simulink subsystem "VehicleBody3DOFLongitudinal"  (R2025b)
settings: Solver=VariableStepAuto  StartTime=0.0  StopTime=10.0  RelTol=1e-3
undefined symbols (not defined in the file): EnvAirTemp, EnvGrvty, PlntVehCGHgtAxl, PlntVehDstCGRearAxl, PlntVehHtchDst, PlntVehHtchHgtAxl, PlntVehHtchLatDst, PlntVehInitVertPos, PlntVehMass
libraries: autolibshared x1
settings Model: ModifiedByFormat=The MathWorks, Inc.  Creator=The MathWorks, Inc.  LastModifiedBy=The MathWorks, Inc.
settings OptimizationCC: ReuseModelBlockBuffer=off
settings DebuggingCC: SubsystemReferenceDiagnosticForUnitTest=warning
settings RTWCC: GPUComputeCapability=3.5

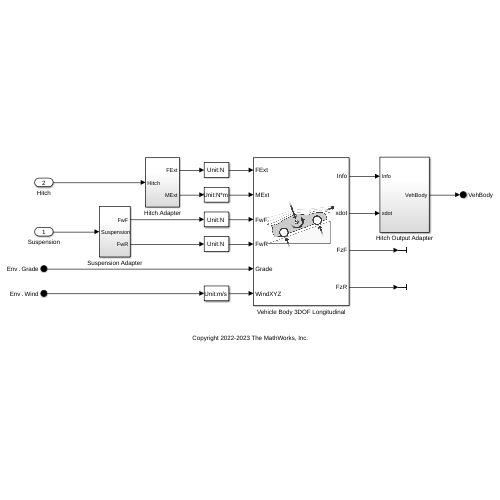
[thumbnail: Simulink's stored preview of the top-level diagram]
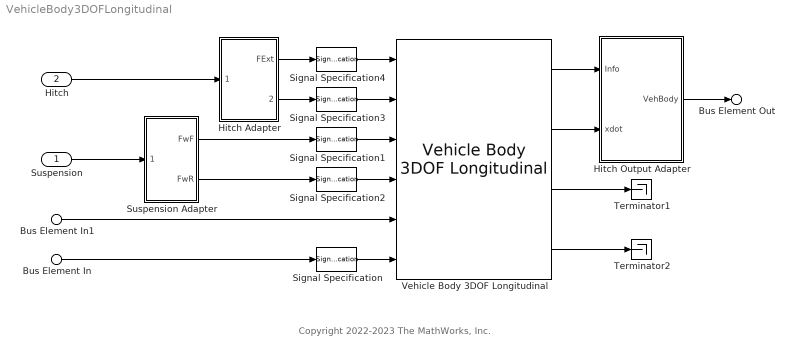
== system VehicleBody3DOFLongitudinal ==
  note: Copyright 2022-2023 The MathWorks, Inc.
  Suspension : Inport
  Hitch : Inport  Port=2
  Bus Element In : Inport  Port=3  PortName=Env  Element=Wind
  Bus Element In1 : Inport  Port=3  PortName=Env  Element=Grade
  Hitch Adapter : Subsystem
  Hitch Output Adapter : Subsystem
  Signal Specification : SignalSpecification  Unit=m/s
  Signal Specification1 : SignalSpecification  Unit=N
  Signal Specification2 : SignalSpecification  Unit=N
  Signal Specification3 : SignalSpecification  Unit=N*m
  Signal Specification4 : SignalSpecification  Unit=N
  Suspension Adapter : Subsystem
  Terminator1 : Terminator
  Terminator2 : Terminator
  Vehicle Body 3DOF Longitudinal : autolibshared/Vehicle Body 3DOF Longitudinal  VariantControl=SL  groundType=Grade angle  aMode=6  extFMode=on  extMMode=on  extTamb=off  NF=PlntVehNumWhlFrntAxl  NR=PlntVehNumWhlRearAxl  m=PlntVehMass  a=PlntVehDstCGFrntAxl  b=PlntVehDstCGRearAxl  h=PlntVehCGHgtAxl  Cd=PlntVehAeroDragCff  Af=PlntVehAeroFrntArea  x_o=PlntVehInitLongPos  xdot_o=PlntVehInitLongVel  Cl=PlntVehAeroLiftCff  z_o=PlntVehInitVertPos-PlntVehCGHgtAxl  zdot_o=0  Iyy=PlntVehPitchMomentInertia  Cpm=PlntVehAeroPitchCff  theta_o=0  q_o=0  FskF=[-50, -1, 0, 2, 3, 52].*1.5e4  dzsF=[-5e-3, -1e-4, 0, .2, .2001, .2051]  FsbF=[-10000 -100 -10 0 10 100 10000]*10  dzdotsF=[-10 -1 -.1 0 .1 1 10]  FskR=[-50, -1, 0, 2, 3, 52].*1e4  dzsR=[-5e-3, -1e-4, 0, .2, .2001, .2051]  FsbR=[-10000 -100 -10 0 10 100 10000]*10  dzdotsR=[-10 -1 -.1 0 .1 1 10]  Pabs=EnvAbsPrs  T=EnvAirTemp  g=EnvGrvty  blkID=0
  Bus Element Out : Outport  PortName=VehBody
  wires:
  Hitch/1 -> Hitch Adapter/1(Hitch)
  Suspension Adapter/2(FwR) -> Signal Specification2/1
  Hitch Adapter/2(MExt) -> Signal Specification3/1
  Hitch Adapter/1(FExt) -> Signal Specification4/1
  Suspension/1 -> Suspension Adapter/1(Suspension)
  Suspension Adapter/1(FwF) -> Signal Specification1/1
  Signal Specification3/1 -> Vehicle Body 3DOF Longitudinal/2
  Signal Specification4/1 -> Vehicle Body 3DOF Longitudinal/1
  Bus Element In/1 -> Signal Specification/1
  Vehicle Body 3DOF Longitudinal/1 -> Hitch Output Adapter/1(Info)
  Vehicle Body 3DOF Longitudinal/3 -> Terminator1/1
  Vehicle Body 3DOF Longitudinal/4 -> Terminator2/1
  Signal Specification/1 -> Vehicle Body 3DOF Longitudinal/6
  Bus Element In1/1 -> Vehicle Body 3DOF Longitudinal/5
  Signal Specification1/1 -> Vehicle Body 3DOF Longitudinal/3
  Signal Specification2/1 -> Vehicle Body 3DOF Longitudinal/4
  Hitch Output Adapter/1(VehBody) -> Bus Element Out/1
  Vehicle Body 3DOF Longitudinal/2 -> Hitch Output Adapter/2(xdot)

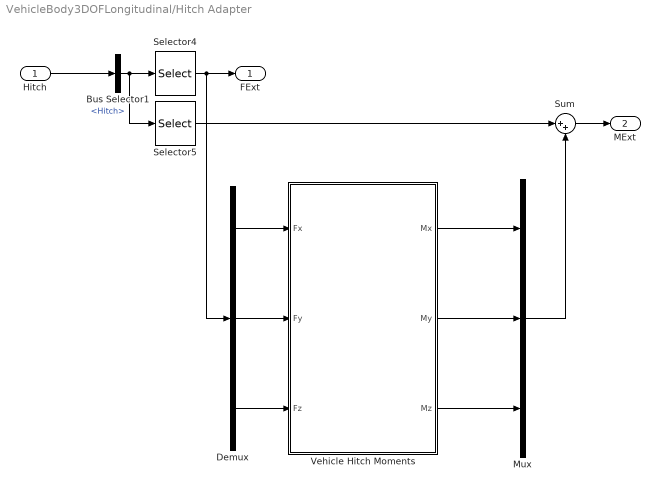
== system VehicleBody3DOFLongitudinal/Hitch Adapter ==
  Hitch : Inport
  Bus Selector1 : BusSelector  OutputSignals=Hitch
  Demux : Demux  Outputs=3
  Mux : Mux  Inputs=3
  Selector4 : Selector  InputPortWidth=6  IndexOptions=Index vector (dialog)  Indices=[1:3]  OutputSizes=1
  Selector5 : Selector  InputPortWidth=6  IndexOptions=Index vector (dialog)  Indices=[4:6]  OutputSizes=1
  Sum : Sum  Inputs=|++
  Vehicle Hitch Moments : Subsystem  mask{h=PlntVehCGHgtAxl, dh=PlntVehHtchDst, hh=PlntVehHtchHgtAxl, hl=PlntVehHtchLatDst}
      mask prompts: h "vdynblks:vehdynTractorBody6Dof:blkPrm_h"; dh "vdynblks:vehdynTractorBody6Dof:blkPrm_dh"; hh "vdynblks:vehdynTractorBody6Dof:blkPrm_hh"; hl "vdynblks:vehdynTractorBody6Dof:blkPrm_hl"
      mask DialogControl h Prompt: Vertical distance from center of mass to axle plane, h [m]:
      mask DialogControl dh Prompt: Longitudinal distance from center of mass to hitch, dh [m]:
      mask DialogControl hh Prompt: Vertical distance from hitch to axle plane, hh [m]:
      mask DialogControl hl Prompt: Lateral distance from geometric centerline to hitch, hl [m]:
  FExt : Outport
  MExt : Outport  Port=2
  wires:
  Selector5/1 -> Sum/1
  Bus Selector1/1 -> Selector5/1, Selector4/1  "<Hitch>"
  Selector4/1 -> FExt/1, Demux/1
  Hitch/1 -> Bus Selector1/1
  Demux/1 -> Vehicle Hitch Moments/1(Fx)
  Demux/2 -> Vehicle Hitch Moments/2(Fy)
  Demux/3 -> Vehicle Hitch Moments/3(Fz)
  Vehicle Hitch Moments/1(Mx) -> Mux/1
  Vehicle Hitch Moments/2(My) -> Mux/2
  Vehicle Hitch Moments/3(Mz) -> Mux/3
  Sum/1 -> MExt/1
  Mux/1 -> Sum/2

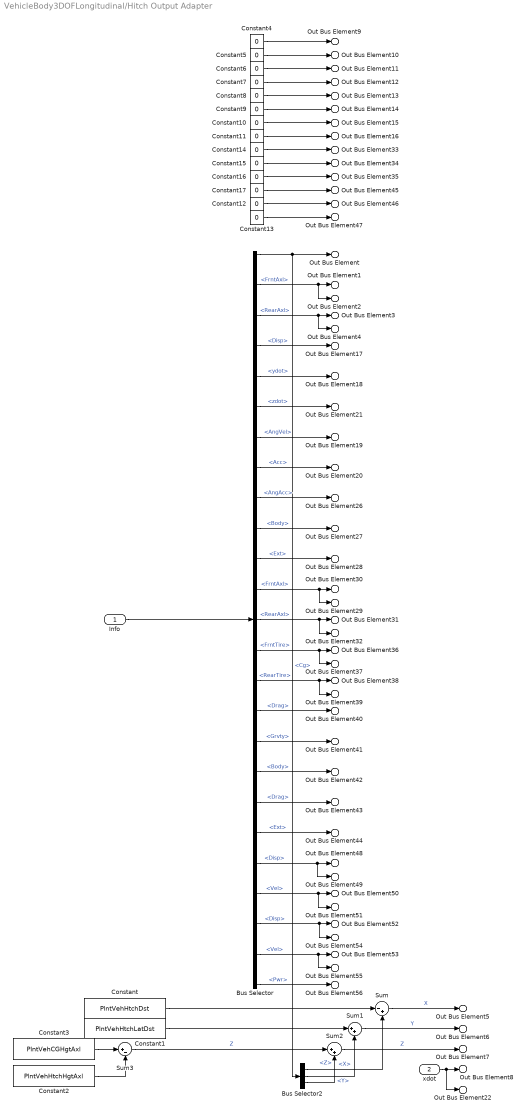
== system VehicleBody3DOFLongitudinal/Hitch Output Adapter ==
  Info : Inport
  xdot : Inport  Port=2
  Bus Selector : BusSelector  OutputSignals=InertFrm.Cg,InertFrm.FrntAxl,InertFrm.RearAxl,BdyFrm.Cg.Disp,BdyFrm.Cg.Vel.ydot,BdyFrm.Cg.Vel.zdot,BdyFrm.Cg.AngVel,BdyFrm.Cg.Acc,BdyFrm.Cg.AngAcc,BdyFrm.Forces.Body,BdyFrm.Forces.Ext,BdyFrm.Forces.FrntAxl,BdyFrm.Forces.RearAxl,BdyFrm.Forces.Tires.FrntTire,BdyFrm.Forces.Tires.RearTire,BdyFrm.Forces.Drag,BdyFrm.Forces.Grvty,BdyFrm.Moments.Body,BdyFrm.Moments.Drag,BdyFrm.Moments.Ext,BdyFrm.FrntAxl.Disp,BdyFrm.FrntAxl.Vel,BdyFrm.RearAxl.Disp,BdyFrm.RearAxl.Vel,BdyFrm.Pwr
  Bus Selector2 : BusSelector  OutputSignals=Disp.X,Disp.Y,Disp.Z
  Constant : Constant  Value=PlntVehHtchDst  SampleTime=-1
  Constant1 : Constant  Value=PlntVehHtchLatDst  SampleTime=-1
  Constant{4..17} (14 alike) : Constant  Value=0  SampleTime=-1
  Constant2 : Constant  Value=PlntVehHtchHgtAxl  SampleTime=-1
  Constant3 : Constant  Value=PlntVehCGHgtAxl  SampleTime=-1
  Sum : Sum  Inputs=|-+
  Sum1 : Sum  Inputs=|++
  Sum2 : Sum  Inputs=|++
  Sum3 : Sum  Inputs=|+-
  Out Bus Element : Outport  PortName=VehBody  Element=InertFrm.Cg
  Out Bus Element1 : Outport  PortName=VehBody  Element=InertFrm.FrntAxl.Lft
  Out Bus Element2 : Outport  PortName=VehBody  Element=InertFrm.FrntAxl.Rght
  Out Bus Element3 : Outport  PortName=VehBody  Element=InertFrm.RearAxl.Lft
  Out Bus Element4 : Outport  PortName=VehBody  Element=InertFrm.RearAxl.Rght
  Out Bus Element5 : Outport  PortName=VehBody  Element=InertFrm.Hitch.Disp.X
  Out Bus Element6 : Outport  PortName=VehBody  Element=InertFrm.Hitch.Disp.Y
  Out Bus Element7 : Outport  PortName=VehBody  Element=InertFrm.Hitch.Disp.Z
  Out Bus Element8 : Outport  PortName=VehBody  Element=InertFrm.Hitch.Vel.Xdot
  Out Bus Element9 : Outport  PortName=VehBody  Element=InertFrm.Hitch.Vel.Ydot
  Out Bus Element10 : Outport  PortName=VehBody  Element=InertFrm.Hitch.Vel.Zdot
  Out Bus Element11 : Outport  PortName=VehBody  Element=InertFrm.Geom.Disp.X
  Out Bus Element12 : Outport  PortName=VehBody  Element=InertFrm.Geom.Disp.Y
  Out Bus Element13 : Outport  PortName=VehBody  Element=InertFrm.Geom.Disp.Z
  Out Bus Element14 : Outport  PortName=VehBody  Element=InertFrm.Geom.Vel.Xdot
  Out Bus Element15 : Outport  PortName=VehBody  Element=InertFrm.Geom.Vel.Ydot
  Out Bus Element16 : Outport  PortName=VehBody  Element=InertFrm.Geom.Vel.Zdot
  Out Bus Element17 : Outport  PortName=VehBody  Element=BdyFrm.Cg.Disp
  Out Bus Element22 : Outport  PortName=VehBody  Element=BdyFrm.Cg.Vel.xdot
  Out Bus Element18 : Outport  PortName=VehBody  Element=BdyFrm.Cg.Vel.ydot
  Out Bus Element21 : Outport  PortName=VehBody  Element=BdyFrm.Cg.Vel.zdot
  Out Bus Element19 : Outport  PortName=VehBody  Element=BdyFrm.Cg.AngVel
  Out Bus Element20 : Outport  PortName=VehBody  Element=BdyFrm.Cg.Acc
  Out Bus Element26 : Outport  PortName=VehBody  Element=BdyFrm.Cg.AngAcc
  Out Bus Element27 : Outport  PortName=VehBody  Element=BdyFrm.Forces.Body
  Out Bus Element28 : Outport  PortName=VehBody  Element=BdyFrm.Forces.Ext
  Out Bus Element29 : Outport  PortName=VehBody  Element=BdyFrm.Forces.FrntAxl.Lft
  Out Bus Element30 : Outport  PortName=VehBody  Element=BdyFrm.Forces.FrntAxl.Rght
  Out Bus Element31 : Outport  PortName=VehBody  Element=BdyFrm.Forces.RearAxl.Lft
  Out Bus Element32 : Outport  PortName=VehBody  Element=BdyFrm.Forces.RearAxl.Rght
  Out Bus Element33 : Outport  PortName=VehBody  Element=BdyFrm.Forces.Hitch.Fx
  Out Bus Element34 : Outport  PortName=VehBody  Element=BdyFrm.Forces.Hitch.Fy
  Out Bus Element35 : Outport  PortName=VehBody  Element=BdyFrm.Forces.Hitch.Fz
  Out Bus Element36 : Outport  PortName=VehBody  Element=BdyFrm.Forces.Tires.FrntTires.Lft
  Out Bus Element37 : Outport  PortName=VehBody  Element=BdyFrm.Forces.Tires.FrntTires.Rght
  Out Bus Element38 : Outport  PortName=VehBody  Element=BdyFrm.Forces.Tires.RearTires.Lft
  Out Bus Element39 : Outport  PortName=VehBody  Element=BdyFrm.Forces.Tires.RearTires.Rght
  Out Bus Element40 : Outport  PortName=VehBody  Element=BdyFrm.Forces.Drag
  Out Bus Element41 : Outport  PortName=VehBody  Element=BdyFrm.Forces.Grvty
  Out Bus Element42 : Outport  PortName=VehBody  Element=BdyFrm.Moments.Body
  Out Bus Element43 : Outport  PortName=VehBody  Element=BdyFrm.Moments.Drag
  Out Bus Element44 : Outport  PortName=VehBody  Element=BdyFrm.Moments.Ext
  Out Bus Element45 : Outport  PortName=VehBody  Element=BdyFrm.Moments.Hitch.Mx
  Out Bus Element46 : Outport  PortName=VehBody  Element=BdyFrm.Moments.Hitch.My
  Out Bus Element47 : Outport  PortName=VehBody  Element=BdyFrm.Moments.Hitch.Mz
  Out Bus Element48 : Outport  PortName=VehBody  Element=BdyFrm.FrntAxl.Lft.Disp
  Out Bus Element50 : Outport  PortName=VehBody  Element=BdyFrm.FrntAxl.Lft.Vel
  Out Bus Element49 : Outport  PortName=VehBody  Element=BdyFrm.FrntAxl.Rght.Disp
  Out Bus Element51 : Outport  PortName=VehBody  Element=BdyFrm.FrntAxl.Rght.Vel
  Out Bus Element52 : Outport  PortName=VehBody  Element=BdyFrm.RearAxl.Lft.Disp
  Out Bus Element53 : Outport  PortName=VehBody  Element=BdyFrm.RearAxl.Lft.Vel
  Out Bus Element54 : Outport  PortName=VehBody  Element=BdyFrm.RearAxl.Rght.Disp
  Out Bus Element55 : Outport  PortName=VehBody  Element=BdyFrm.RearAxl.Rght.Vel
  Out Bus Element56 : Outport  PortName=VehBody  Element=BdyFrm.Pwr
  wires:
  Bus Selector/7 -> Out Bus Element19/1  "<AngVel>"
  Bus Selector/9 -> Out Bus Element26/1  "<AngAcc>"
  Bus Selector/8 -> Out Bus Element20/1  "<Acc>"
  Bus Selector/5 -> Out Bus Element18/1  "<ydot>"
  Bus Selector/4 -> Out Bus Element17/1  "<Disp>"
  Bus Selector/24 -> Out Bus Element53/1, Out Bus Element55/1  "<Vel>"
  Bus Selector/23 -> Out Bus Element54/1, Out Bus Element52/1  "<Disp>"
  Bus Selector/22 -> Out Bus Element50/1, Out Bus Element51/1  "<Vel>"
  Bus Selector/21 -> Out Bus Element48/1, Out Bus Element49/1  "<Disp>"
  Bus Selector/25 -> Out Bus Element56/1  "<Pwr>"
  Bus Selector/20 -> Out Bus Element44/1  "<Ext>"
  Bus Selector/19 -> Out Bus Element43/1  "<Drag>"
  Bus Selector/18 -> Out Bus Element42/1  "<Body>"
  Bus Selector/17 -> Out Bus Element41/1  "<Grvty>"
  Bus Selector/16 -> Out Bus Element40/1  "<Drag>"
  Bus Selector/15 -> Out Bus Element38/1, Out Bus Element39/1  "<RearTire>"
  Bus Selector/14 -> Out Bus Element37/1, Out Bus Element36/1  "<FrntTire>"
  Bus Selector/13 -> Out Bus Element32/1, Out Bus Element31/1  "<RearAxl>"
  Bus Selector/12 -> Out Bus Element30/1, Out Bus Element29/1  "<FrntAxl>"
  Bus Selector/11 -> Out Bus Element28/1  "<Ext>"
  Bus Selector/10 -> Out Bus Element27/1  "<Body>"
  Bus Selector/3 -> Out Bus Element4/1, Out Bus Element3/1  "<RearAxl>"
  Bus Selector/2 -> Out Bus Element1/1, Out Bus Element2/1  "<FrntAxl>"
  Bus Selector/1 -> Bus Selector2/1, Out Bus Element/1  "<Cg>"
  Info/1 -> Bus Selector/1
  Constant/1 -> Sum/1
  Sum3/1 -> Sum2/1  "Z"
  Constant3/1 -> Sum3/1
  Sum2/1 -> Out Bus Element7/1  "Z"
  Constant2/1 -> Sum3/2
  Sum/1 -> Out Bus Element5/1  "X"
  Sum1/1 -> Out Bus Element6/1  "Y"
  Constant1/1 -> Sum1/1
  xdot/1 -> Out Bus Element22/1, Out Bus Element8/1
  Constant4/1 -> Out Bus Element9/1
  Constant5/1 -> Out Bus Element10/1
  Constant6/1 -> Out Bus Element11/1
  Constant7/1 -> Out Bus Element12/1
  Constant8/1 -> Out Bus Element13/1
  Constant9/1 -> Out Bus Element14/1
  Constant10/1 -> Out Bus Element15/1
  Constant11/1 -> Out Bus Element16/1
  Constant14/1 -> Out Bus Element33/1
  Constant15/1 -> Out Bus Element34/1
  Constant16/1 -> Out Bus Element35/1
  Constant17/1 -> Out Bus Element45/1
  Constant12/1 -> Out Bus Element46/1
  Constant13/1 -> Out Bus Element47/1
  Bus Selector/6 -> Out Bus Element21/1  "<zdot>"
  Bus Selector2/1 -> Sum/2  "<X>"
  Bus Selector2/2 -> Sum1/2  "<Y>"
  Bus Selector2/3 -> Sum2/2  "<Z>"

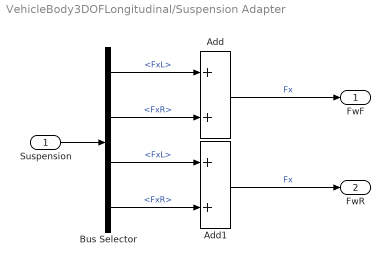
== system VehicleBody3DOFLongitudinal/Suspension Adapter ==
  Suspension : Inport
  Add : Sum
  Add1 : Sum
  Bus Selector : BusSelector  OutputSignals=FrntSusp.FrntSuspWheel.Wheels.Fx.FxL,FrntSusp.FrntSuspWheel.Wheels.Fx.FxR,RearSusp.RearSuspWheel.Wheels.Fx.FxL,RearSusp.RearSuspWheel.Wheels.Fx.FxR
  FwF : Outport
  FwR : Outport  Port=2
  wires:
  Bus Selector/4 -> Add1/2  "<FxR>"
  Bus Selector/3 -> Add1/1  "<FxL>"
  Bus Selector/2 -> Add/2  "<FxR>"
  Bus Selector/1 -> Add/1  "<FxL>"
  Add/1 -> FwF/1  "Fx"
  Add1/1 -> FwR/1  "Fx"
  Suspension/1 -> Bus Selector/1

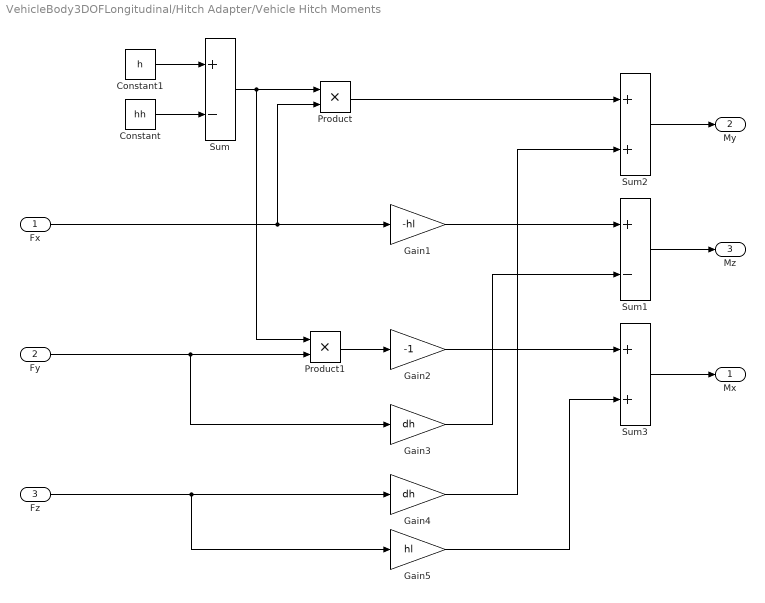
== system VehicleBody3DOFLongitudinal/Hitch Adapter/Vehicle Hitch Moments ==
  Fx : Inport
  Fy : Inport  Port=2
  Fz : Inport  Port=3
  Constant : Constant  Value=hh  SampleTime=-1
  Constant1 : Constant  Value=h  SampleTime=-1
  Gain1 : Gain  Gain=-hl
  Gain2 : Gain  Gain=-1
  Gain3 : Gain  Gain=dh
  Gain4 : Gain  Gain=dh
  Gain5 : Gain  Gain=hl
  Product : Product
  Product1 : Product
  Sum : Sum  Inputs=+-
  Sum1 : Sum  Inputs=+-
  Sum2 : Sum
  Sum3 : Sum
  Mx : Outport
  My : Outport  Port=2
  Mz : Outport  Port=3
  wires:
  Fy/1 -> Gain3/1, Product1/2
  Product1/1 -> Gain2/1
  Sum/1 -> Product1/1, Product/1
  Product/1 -> Sum2/1
  Constant1/1 -> Sum/1
  Gain3/1 -> Sum1/2
  Fx/1 -> Product/2, Gain1/1
  Fz/1 -> Gain5/1, Gain4/1
  Sum2/1 -> My/1
  Constant/1 -> Sum/2
  Gain1/1 -> Sum1/1
  Gain4/1 -> Sum2/2
  Gain5/1 -> Sum3/2
  Gain2/1 -> Sum3/1
  Sum1/1 -> Mz/1
  Sum3/1 -> Mx/1
